simulink model "exercitiul2"  (R2021b)
settings: Solver=VariableStepAuto  StartTime=0.0  StopTime=10.0  RelTol=1e-3
undefined symbols (not defined in the file or in its folder): A, B, C, D, x0
libraries: simulink x4
settings Model: Creator=george.tudor1906  LastModifiedBy=george.tudor1906

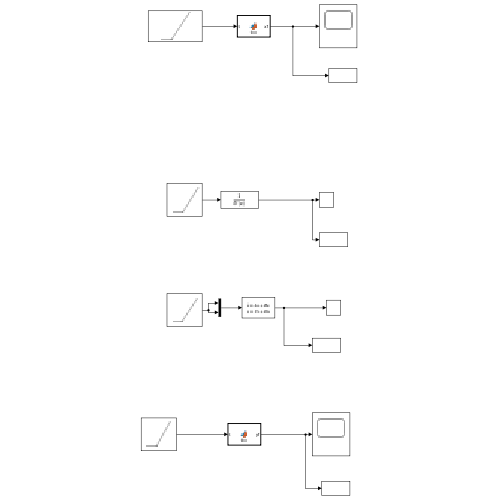
[thumbnail: Simulink's stored preview of the top-level diagram]
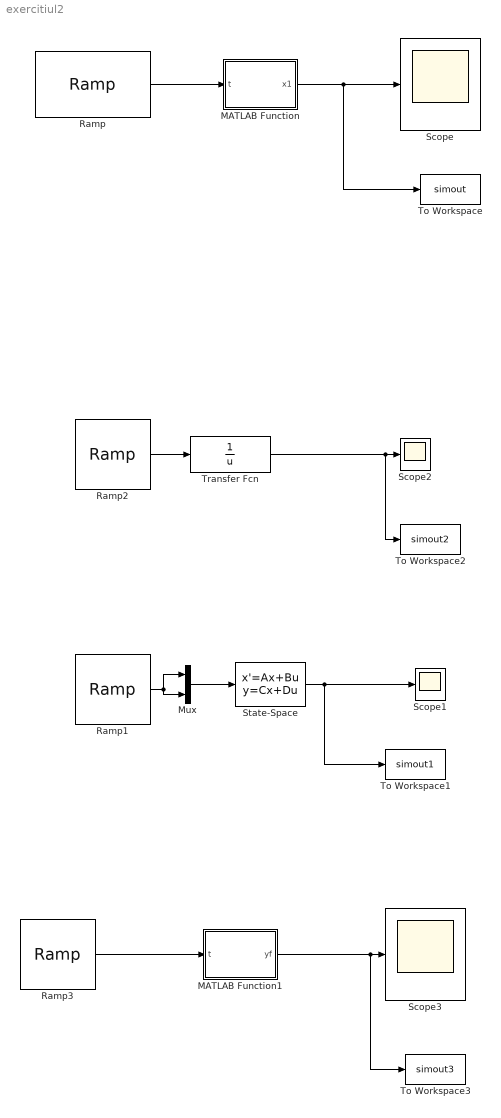
== system exercitiul2 ==
  MATLAB Function : MATLAB Function  TreatAsAtomicUnit=on
  MATLAB Function1 : MATLAB Function  TreatAsAtomicUnit=on
  Mux : Mux  Inputs=2
  Ramp{,1..3} (4 alike) : simulink/Sources/Ramp  slope=1  start=0  InitialOutput=0
  Scope{,1..3} (4 alike) : Scope
  State-Space : StateSpace  A=A  B=B  C=C  D=D  InitialCondition=x0
  To Workspace : ToWorkspace  VariableName=simout  SaveFormat=Timeseries  SampleTime=-1
  To Workspace1 : ToWorkspace  VariableName=simout1  SaveFormat=Timeseries  SampleTime=-1
  To Workspace2 : ToWorkspace  VariableName=simout2  SaveFormat=Timeseries  SampleTime=-1
  To Workspace3 : ToWorkspace  VariableName=simout3  SaveFormat=Timeseries  SampleTime=-1
  Transfer Fcn : TransferFcn  Denominator=u
  wires:
  Transfer Fcn/1 -> To Workspace2/1, Scope2/1
  State-Space/1 -> To Workspace1/1, Scope1/1
  Ramp3/1 -> MATLAB Function1/1(t)
  Ramp2/1 -> Transfer Fcn/1
  MATLAB Function/1(x1) -> To Workspace/1, Scope/1
  MATLAB Function1/1(yf) -> To Workspace3/1, Scope3/1
  Ramp/1 -> MATLAB Function/1(t)
  Mux/1 -> State-Space/1
  Ramp1/1 -> Mux/2, Mux/1

== matlab function exercitiul2/MATLAB Function ==
  data: t input; x1 output
function x1 = fcn(t)
  x1 = [exp(-t); exp(-t)*(cos(10*t) - sin(10*t)/10) - exp(-t) + (101*sin(10*t)*exp(-t))/10;(sin(10*t)*exp(-t))/10 - exp(-t)*(cos(10*t))]; 
end

== matlab function exercitiul2/MATLAB Function1 ==
  data: t input; yf output
function yf = fcn(t)
  yf = (101*sin(10*t)*exp(-t))/10 - 2*exp(-t);
end
